simulink model "task_E1_mod"  (R2018a)
settings: Solver=ode45  StartTime=0.0  StopTime=10.0  RelTol=1e-3  EnableMultiTasking=on
values from neighbouring files (symbols this model uses):
  b = 2    [task_E1_scr.m]    (also in task_E_scr.m)
  nmax = 1.1    [task_E1_scr.m]    (also in task_E_scr.m; task_F1_scr.m; task_F_scr.m; task_G_scr.m)
  nmin = 0.9    [task_E1_scr.m]    (also in task_E_scr.m; task_F1_scr.m; task_F_scr.m; task_G_scr.m)
  nois = 1; sim('task_E1_mod',10)    [task_E1_scr.m]    (also in task_E_scr.m; task_F1_scr.m = 1; task_F_scr.m = 1; sim('task_F_mod',8); task_G_scr.m = 1; sim('task_G_mod',15))
settings Model: Creator=Yurii  LastModifiedBy=Master
settings DataIOCC: LimitDataPoints=on  SaveFormat=Array
settings OptimizationCC: LifeSpan=inf
settings DebuggingCC: UnderspecifiedInitializationDetection=Classic  MergeDetectMultiDrivingBlocksExec=none  SolverPrmCheckMsg=warning  SFUnexpectedBacktrackingDiag=warning  SFNoUnconditionalDefaultTransitionDiag=warning  SFExecutionAtInitializationDiag=none
settings HardwareCC: ProdBitPerPointer=32  ProdBitPerSizeT=32  ProdBitPerPtrDiffT=32  ProdLargestAtomicFloat=None  ProdIntDivRoundTo=Undefined  ProdEndianess=Unspecified  ProdWordSize=32  ProdHWDeviceType=32-bit Generic
settings ModelReferenceCC: PropagateSignalLabelsOutOfModel=off
settings CodeAppCC: StateflowObjectComments=on
settings GRTTargetCC: TargetLangStandard=C89/C90 (ANSI)  GeneratePreprocessorConditionals=Disable all
settings ConfigComp: CovMetricSettings=dw  CovHtmlReporting=on  CovSaveCumulativeToWorkspaceVar=on  CovSaveSingleToWorkspaceVar=on  CovExternalEMLEnable=off

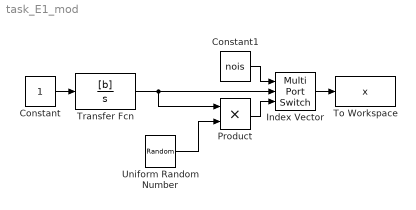
== system task_E1_mod ==
  Constant : Constant
  Constant1 : Constant  Value=nois
  Index Vector : MultiPortSwitch  DataPortOrder=Zero-based contiguous  Inputs=2  zeroidx=on
  Product : Product
  To Workspace : ToWorkspace  VariableName=x  SaveFormat=Timeseries  SampleTime=-1
  Transfer Fcn : TransferFcn  Numerator=[b]  Denominator=[1 0]
  Uniform Random Number : UniformRandomNumber  Minimum=nmin  Maximum=nmax  SampleTime=0.1
  wires:
  Constant/1 -> Transfer Fcn/1
  Uniform Random Number/1 -> Product/2
  Transfer Fcn/1 -> Product/1, Index Vector/2
  Product/1 -> Index Vector/3
  Index Vector/1 -> To Workspace/1
  Constant1/1 -> Index Vector/1
